simulink model "Model_nie_liniowy_zapiete_sprzerzenie"  (R2017a)
settings: Solver=ode45  StartTime=0.0  StopTime=20  FixedStep=0.01  MaxStep=0.0001  RelTol=1e-5  EnableMultiTasking=on
values from neighbouring files (symbols this model uses):
  L = lqr(A, B, Q, R)    [Linearyzacja_ramienia_robota.m]    (also in filtr_kalmana_Mateusz.m = (eye(4) - K*C_D)*B_D; sciaga.m = lqr(A,B,Q,R))
libraries: simulink x4
settings Model: Creator=kss  LastModifiedBy=Szwank
settings SolverCC: MaxConsecutiveZCs=100000  ZeroCrossControl=EnableAll  SolverResetMethod=Robust
settings OptimizationCC: LifeSpan=inf
settings DebuggingCC: SFUnexpectedBacktrackingDiag=warning  SFNoUnconditionalDefaultTransitionDiag=warning  SFExecutionAtInitializationDiag=none
settings GRTTargetCC: TargetLangStandard=C89/C90 (ANSI)  GeneratePreprocessorConditionals=Disable all
settings ConfigComp: CovMetricSettings=dw  CovHtmlReporting=on  CovSaveCumulativeToWorkspaceVar=on  CovSaveSingleToWorkspaceVar=on  CovExternalEMLEnable=off

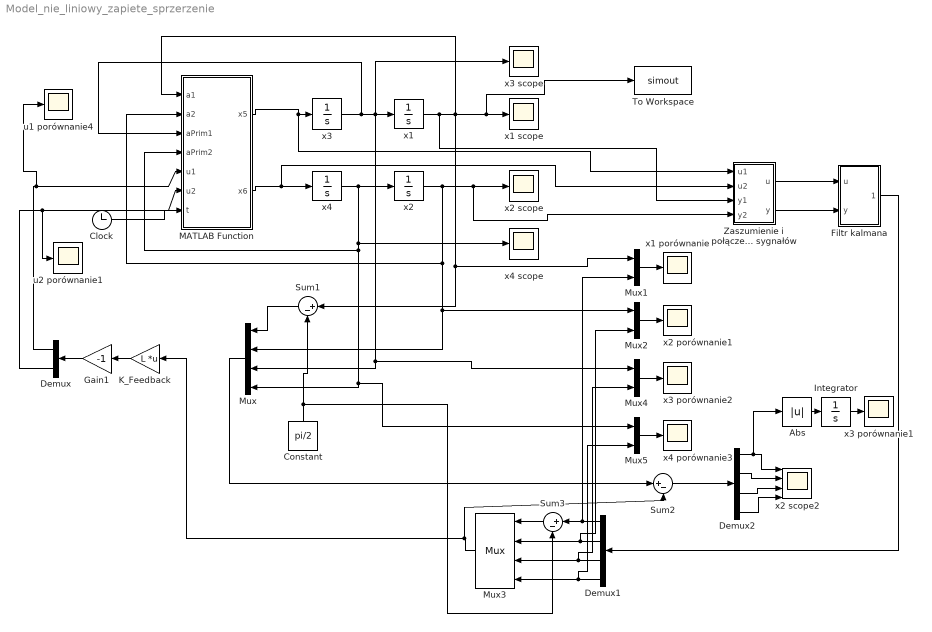
== system Model_nie_liniowy_zapiete_sprzerzenie ==
  Abs : Abs
  Clock : Clock
  Constant : Constant  Value=pi/2
  Demux : Demux  Outputs=2
  Demux1 : Demux
  Demux2 : Demux
  Filtr kalmana : Subsystem
  Gain1 : Gain  Gain=-1
  Integrator : Integrator
  K_Feedback : Gain  Gain=L  Multiplication=Matrix(K*u)
  MATLAB Function : MATLAB Function  TreatAsAtomicUnit=on
  Mux : Mux
  Mux{1..2,4..5} (4 alike) : Mux  Inputs=2
  Mux3 : Mux
      settings: DisplayOption=signals
  Sum1 : Sum  Inputs=|+-
  Sum2 : Sum  Inputs=|+-
  Sum3 : Sum  Inputs=|+-
  To Workspace : ToWorkspace  VariableName=simout  SaveFormat=Timeseries  SampleTime=-1
  Zaszumienie i połączenie sygnałów : Subsystem
  u1 porównanie4 : Scope
  u2 porównanie1 : Scope
  x1 : Integrator  InitialCondition=(pi/2)-0.3  AbsoluteTolerance=1e-5
  x1 porównanie : Scope
  x1 scope : Scope
  x2 : Integrator  InitialCondition=0.3  AbsoluteTolerance=1e-5
  x2 porównanie1 : Scope
  x2 scope : Scope
  x2 scope2 : Scope  NumInputPorts=4
  x3 : Integrator  AbsoluteTolerance=1e-5
  x3 porównanie1 : Scope
  x3 porównanie2 : Scope
  x3 scope : Scope
  x4 : Integrator  AbsoluteTolerance=1e-5
  x4 porównanie3 : Scope
  x4 scope : Scope
  wires:
  MATLAB Function/1(x5) -> Zaszumienie i połączenie sygnałów/1(u1), x3/1
  MATLAB Function/2(x6) -> Zaszumienie i połączenie sygnałów/2(u2), x4/1
  x3/1 -> MATLAB Function/3(aPrim1), x3 scope/1, Mux4/1, Mux/3, x1/1
  x4/1 -> x4 scope/1, Mux5/1, Mux/4, MATLAB Function/4(aPrim2), x2/1
  x2/1 -> Zaszumienie i połączenie sygnałów/4(y2), x2 scope/1, Mux2/1, Mux/2, MATLAB Function/2(a2)
  Sum1/1 -> Mux/1
  Constant/1 -> Sum3/2, Sum1/2
  Demux1/1 -> Mux1/2, Sum3/1
  Sum3/1 -> Mux3/1
  Demux1/2 -> Mux2/2, Mux3/2
  Demux1/3 -> Mux4/2, Mux3/3
  Demux1/4 -> Mux5/2, Mux3/4
  Filtr kalmana/1(Out1) -> Demux1/1
  Zaszumienie i połączenie sygnałów/1(u) -> Filtr kalmana/1(u)
  Zaszumienie i połączenie sygnałów/2(y) -> Filtr kalmana/2(y)
  Mux1/1 -> x1 porównanie/1
  Mux3/1 -> K_Feedback/1, Sum2/2
  Mux/1 -> Sum2/1
  x1/1 -> Zaszumienie i połączenie sygnałów/3(y1), Sum1/1, Mux1/1, To Workspace/1, x1 scope/1, MATLAB Function/1(a1)
  K_Feedback/1 -> Gain1/1
  Demux/1 -> u1 porównanie4/1, MATLAB Function/5(u1)
  Demux/2 -> MATLAB Function/6(u2), u2 porównanie1/1
  Gain1/1 -> Demux/1
  Mux2/1 -> x2 porównanie1/1
  Mux4/1 -> x3 porównanie2/1
  Mux5/1 -> x4 porównanie3/1
  Clock/1 -> MATLAB Function/7(t)
  Sum2/1 -> Demux2/1
  Demux2/2 -> x2 scope2/2
  Demux2/3 -> x2 scope2/3
  Demux2/4 -> x2 scope2/4
  Demux2/1 -> Abs/1, x2 scope2/1
  Integrator/1 -> x3 porównanie1/1
  Abs/1 -> Integrator/1

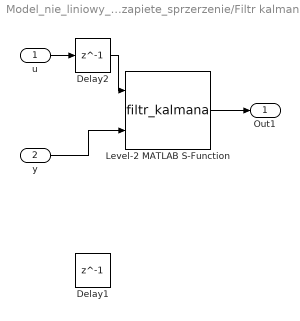
== system Model_nie_liniowy_zapiete_sprzerzenie/Filtr kalmana ==
  u : Inport
  y : Inport  Port=2
  Delay1 : Delay  DelayLength=1  InitialCondition=[pi/2-0.3;0.3]  SampleTime=0.0001
  Delay2 : Delay  DelayLength=1  SampleTime=0.0001
  Level-2 MATLAB S-Function : M-S-Function  FunctionName=filtr_kalmana  Parameters=[(pi/2)-0.3; 0.3; 0; 0]
  Out1 : Outport
  wires:
  Level-2 MATLAB S-Function/1 -> Out1/1
  u/1 -> Delay2/1
  Delay2/1 -> Level-2 MATLAB S-Function/1
  y/1 -> Level-2 MATLAB S-Function/2

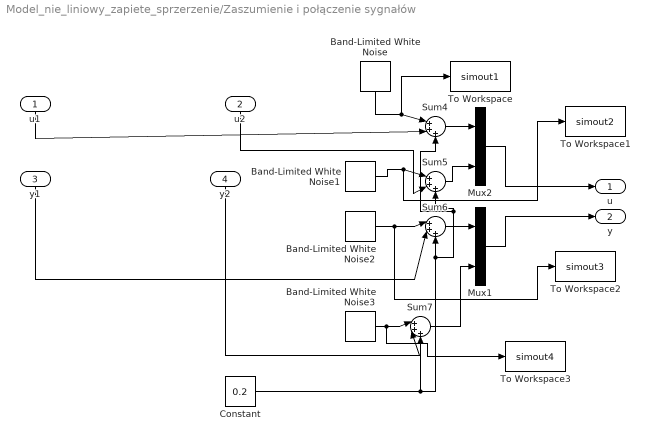
== system Model_nie_liniowy_zapiete_sprzerzenie/Zaszumienie i połączenie sygnałów ==
  u1 : Inport
  u2 : Inport  Port=2
  y1 : Inport  Port=3
  y2 : Inport  Port=4
  Band-Limited White Noise : simulink/Sources/Band-Limited White Noise  Cov=[0.001]  Ts=0.01  seed=[11111]
  Band-Limited White Noise1 : simulink/Sources/Band-Limited White Noise  Cov=[0.001]  Ts=0.01  seed=[22345]
  Band-Limited White Noise2 : simulink/Sources/Band-Limited White Noise  Cov=[0.001]  Ts=0.01  seed=[145633]
  Band-Limited White Noise3 : simulink/Sources/Band-Limited White Noise  Cov=[0.001]  Ts=0.01  seed=[521238]
  Constant : Constant  Value=0.2
  Mux1 : Mux  Inputs=2
  Mux2 : Mux  Inputs=2
  Sum{4..7} (4 alike) : Sum  Inputs=|+++
  To Workspace : ToWorkspace  VariableName=simout1  SaveFormat=Timeseries  SampleTime=-1
  To Workspace1 : ToWorkspace  VariableName=simout2  SaveFormat=Timeseries  SampleTime=-1
  To Workspace2 : ToWorkspace  VariableName=simout3  SaveFormat=Timeseries  SampleTime=-1
  To Workspace3 : ToWorkspace  VariableName=simout4  SaveFormat=Timeseries  SampleTime=-1
  u : Outport
  y : Outport  Port=2
  wires:
  u1/1 -> Sum4/2
  y2/1 -> Sum7/2
  Sum5/1 -> Mux2/2
  Sum7/1 -> Mux1/2
  Mux2/1 -> u/1
  Mux1/1 -> y/1
  Sum4/1 -> Mux2/1
  Sum6/1 -> Mux1/1
  u2/1 -> Sum5/2
  y1/1 -> Sum6/2
  Band-Limited White Noise/1 -> To Workspace/1, Sum4/1
  Band-Limited White Noise1/1 -> To Workspace1/1, Sum5/1
  Band-Limited White Noise2/1 -> To Workspace2/1, Sum6/1
  Band-Limited White Noise3/1 -> To Workspace3/1, Sum7/1
  Constant/1 -> Sum4/3, Sum5/3, Sum6/3, Sum7/3

== matlab function Model_nie_liniowy_zapiete_sprzerzenie/MATLAB Function ==
  data: a1 input; a2 input; aPrim1 input; aPrim2 input; u1 input; u2 input; x5 output; x6 output; t input
function [x5,x6] = fcn(a1,a2,aPrim1,aPrim2,u1,u2,t)
m1 = 2; m2 = 1; l1 = 1.5; l2 = 1; lc1 = l1/2; lc2 = l2/2; J1 = (m1*l1^2)/3; J2 = (m2*l2^2)/3; g = 9.81;
H11 = m1*lc1^2 + J1 + m2*(l1^2 + lc2^2 + 2*l1*l2*cos(a2)) + J2;
H12  = m2*l1*lc2*cos(a2) + m2*lc2^2 + J2;
H21 = H12;
H22 = m2*lc2^2 + J2;
h = m2*l1*lc2*sin(a2);
g1 = m1*lc1*g*cos(a1) + m2*g*(lc2*cos(a1+a2)+l1*cos(a1));
g2 = m2*lc2*g*cos(a1+a2);
H = [H11 H12; H21 H22];
H2 = inv(H);
Z = [0.2*sin(t);0.5*cos(t)];

J = [-h*aPrim2, -h*aPrim1-h*aPrim2; h*aPrim1,0];
M = [g1;g2];
U = [u1;u2];
%rozwikłanie 
Roz = -1*H2*J*[aPrim1; aPrim2] -1*H2*M + H2*U + H2 * Z; 
x5 = Roz(1);
x6 = Roz(2);
% x5 = (200*T1 - 200*T2 + (2943*cos(x1 + 2*x2))/2 - (8829*cos(x1))/2 + 150*x3^2*sin(x2) + 150*x4^2*sin(x2) + 225*x3^2*sin(2*x2) - 23544*J2*cos(x1) - 600*T2*cos(x2) + 800*J2*T1 - 800*J2*T2 + 300*x3*x4*sin(x2) + 600*J2*x3^2*sin(x2) + 600*J2*x4^2*sin(x2) + 1200*J2*x3*x4*sin(x2))/(25*(8*J1 + 108*J2 - 9*cos(2*x2) + 32*J1*J2 + 18));
% x6 = -(400*T1 - 5800*T2 - 17658*cos(x1 - x2) + 2943*cos(x1 + 2*x2) + 8829*cos(x1 + x2) - 8829*cos(x1) + 4350*x3^2*sin(x2) + 300*x4^2*sin(x2) + 7848*J1*cos(x1 + x2) + 900*x3^2*sin(2*x2) + 450*x4^2*sin(2*x2) - 47088*J2*cos(x1) + 1200*T1*cos(x2) - 2400*T2*cos(x2) - 1600*J1*T2 + 1600*J2*T1 - 1600*J2*T2 + 600*x3*x4*sin(x2) + 1200*J1*x3^2*sin(x2) + 1200*J2*x3^2*sin(x2) + 1200*J2*x4^2*sin(x2) + 900*x3*x4*sin(2*x2) + 2400*J2*x3*x4*sin(x2))/(50*(8*J1 + 108*J2 - 9*cos(2*x2) + 32*J1*J2 + 18));

%y = u;
